simulink model "model_d"  (R2021a)
settings: Solver=VariableStepAuto  StartTime=0.0  StopTime=T  RelTol=1e-3
values from neighbouring files (symbols this model uses):
  A = simplify([A_nl_theta A_nl_x A_nl_theta1 A_nl_x1])    [Exercise.m]    (also in Final_Control.m = double(subs(subs(Ap, parameters, values), parameters, values; Kinematics.m = simplify([A_theta, A_x, A_theta1, A_x1]); control.m = double(subs(Ap, parameters, values)); control_d.m = double(subs(Ap, parameters, values)))
  Ad = sys_d.a    [Final_Control.m]    (also in control_d.m)
  B = subs(B_nl, {theta, theta1, x, x1}, {0, 0, 0, 0})    [Exercise.m]    (also in Final_Control.m = double(subs(subs(Bp, parameters, values), parameters, values; Kinematics.m = simplify(subs(Bnl, vars, point)); control.m = double(subs(Bp, parameters, values)); control_d.m = double(subs(Bp, parameters, values)))
  Bd = sys_d.b    [Final_Control.m]    (also in control_d.m)
  C = eye(4)    [Final_Control.m]    (also in control.m = [1 0 0 0; 0 1 0 0]; control_d.m = [0 1 0 0])
  Cd = sys_d.c    [Final_Control.m]    (also in control_d.m)
  K = dlqr(Ad, Bd, Q, R)    [Final_Control.m]    (also in control.m = lqr(A, B, Q, R); control_d.m = acker(Ad, Bd, poles))
  Kobs = acker(Ad', Cd', poles*0.1)    [control_d.m]
  pt = cell2mat(point)'    [Final_Control.m]    (also in control.m; control_d.m)
  r = [pi/2;0;0;0]    [Final_Control.m]    (also in control.m; control_d.m)
  Ts = 1/100    (= 0.01)    [Final_Control.m]    (also in control_d.m = 0.1)
  x0 = X0 - pt    [Final_Control.m]    (also in control.m; control_d.m)
settings Model: Creator=Usuario  LastModifiedBy=Usuario

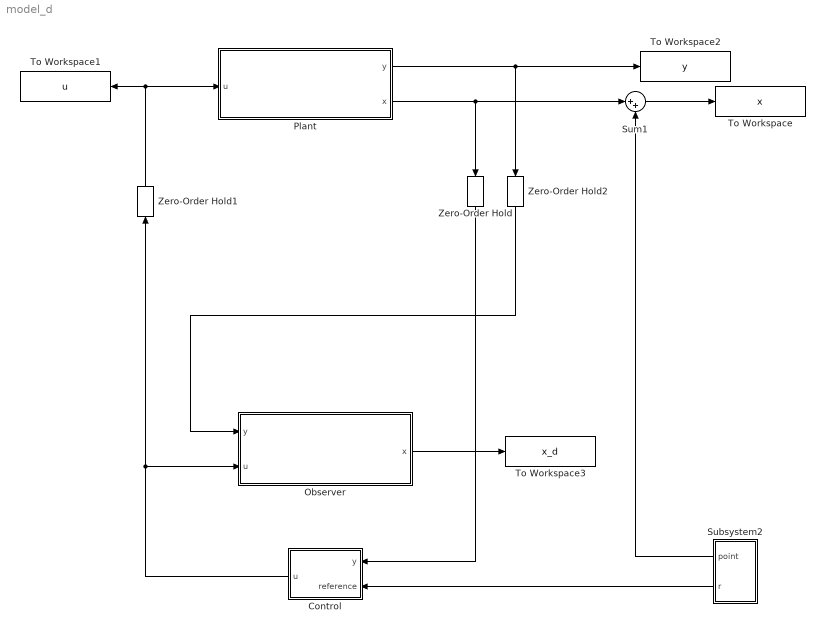
== system model_d ==
  Control : Subsystem
  Observer : Subsystem
  Plant : Subsystem
  Subsystem2 : Subsystem
  Sum1 : Sum  Inputs=|++
  To Workspace : ToWorkspace  VariableName=x  SaveFormat=Timeseries  SampleTime=-1
  To Workspace1 : ToWorkspace  VariableName=u  SaveFormat=Timeseries  SampleTime=-1
  To Workspace2 : ToWorkspace  VariableName=y  SaveFormat=Timeseries  SampleTime=-1
  To Workspace3 : ToWorkspace  VariableName=x_d  SaveFormat=Timeseries  SampleTime=-1
  Zero-Order Hold : ZeroOrderHold  SampleTime=Ts
  Zero-Order Hold1 : ZeroOrderHold  SampleTime=Ts
  Zero-Order Hold2 : ZeroOrderHold  SampleTime=Ts
  wires:
  Plant/1(y) -> Zero-Order Hold2/1, To Workspace2/1
  Sum1/1 -> To Workspace/1
  Subsystem2/1(point) -> Sum1/2
  Subsystem2/2(r) -> Control/2(reference)
  Plant/2(x) -> Sum1/1, Zero-Order Hold/1
  Zero-Order Hold1/1 -> Plant/1(u), To Workspace1/1
  Control/1(u) -> Zero-Order Hold1/1, Observer/2(u)
  Zero-Order Hold2/1 -> Observer/1(y)
  Observer/1(x) -> To Workspace3/1
  Zero-Order Hold/1 -> Control/1(y)

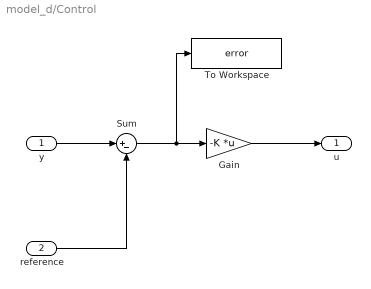
== system model_d/Control ==
  y : Inport
  reference : Inport  Port=2
  Gain : Gain  Gain=-K  Multiplication=Matrix(K*u)
  Sum : Sum  Inputs=|+-
  To Workspace : ToWorkspace  VariableName=error  SaveFormat=Timeseries  SampleTime=-1
  u : Outport
  wires:
  Gain/1 -> u/1
  Sum/1 -> To Workspace/1, Gain/1
  y/1 -> Sum/1
  reference/1 -> Sum/2

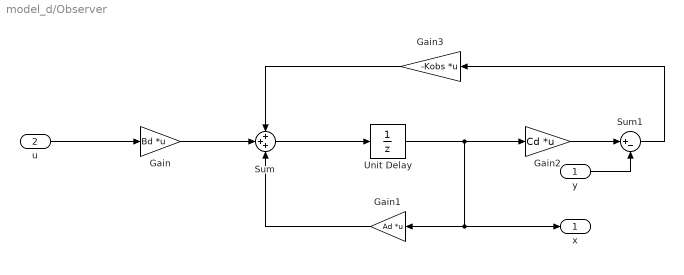
== system model_d/Observer ==
  y : Inport
  u : Inport  Port=2
  Gain : Gain  Gain=Bd  Multiplication=Matrix(K*u)
  Gain1 : Gain  Gain=Ad  Multiplication=Matrix(K*u)
  Gain2 : Gain  Gain=Cd  Multiplication=Matrix(K*u)
  Gain3 : Gain  Gain=-Kobs  Multiplication=Matrix(K*u)
  Sum : Sum  Inputs=+++
  Sum1 : Sum  Inputs=|+-
  Unit Delay : UnitDelay  SampleTime=Ts  HasFrameUpgradeWarning=on
  x : Outport
  wires:
  u/1 -> Gain/1
  Sum/1 -> Unit Delay/1
  Unit Delay/1 -> Gain1/1, x/1, Gain2/1
  Gain2/1 -> Sum1/1
  y/1 -> Sum1/2
  Gain/1 -> Sum/2
  Gain1/1 -> Sum/3
  Sum1/1 -> Gain3/1
  Gain3/1 -> Sum/1

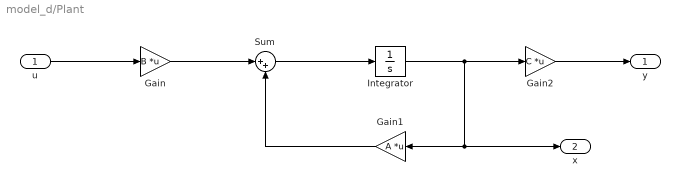
== system model_d/Plant ==
  u : Inport
  Gain : Gain  Gain=B  Multiplication=Matrix(K*u)
  Gain1 : Gain  Gain=A  Multiplication=Matrix(K*u)
  Gain2 : Gain  Gain=C  Multiplication=Matrix(K*u)
  Integrator : Integrator  InitialCondition=x0
  Sum : Sum  Inputs=|++
  y : Outport
  x : Outport  Port=2
  wires:
  Gain/1 -> Sum/1
  Integrator/1 -> Gain2/1, x/1, Gain1/1
  Sum/1 -> Integrator/1
  Gain1/1 -> Sum/2
  u/1 -> Gain/1
  Gain2/1 -> y/1

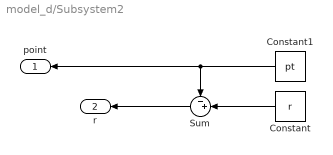
== system model_d/Subsystem2 ==
  Constant : Constant  Value=r
  Constant1 : Constant  Value=pt
  Sum : Sum  Inputs=-+|
  point : Outport
  r : Outport  Port=2
  wires:
  Constant1/1 -> point/1, Sum/1
  Constant/1 -> Sum/2
  Sum/1 -> r/1
